simulink model "PID_nn"  (R2018a)
settings: Solver=ode45  StartTime=0.0  StopTime=300  FixedStep=0.001  RelTol=1e-3
undefined symbols (not defined in the file): now
libraries: neural x1, simulink x1
settings Model: Creator=DELL  LastModifiedBy=DELL
settings DataIOCC: ReturnWorkspaceOutputs=on
settings SFSimCC: SimUseLocalCustomCode=on
settings RTWCC: RTWUseLocalCustomCode=on

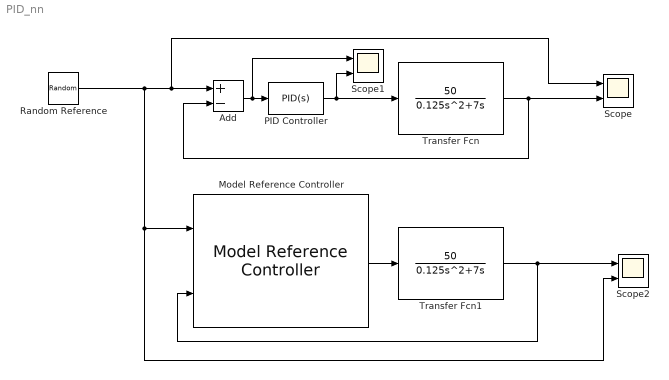
== system PID_nn ==
  Add : Sum  Inputs=+-
  Model Reference Controller : neural/Control Systems/Model Reference Controller  Nrc=2  Nic=1  Njc=2  IW_y=[0.76926837281400406443 1.0491724930046117947;-1.5649571917305367119 -1.6262067418210035541;0.10169527028746853936 -2.2807887773906636575;-0.18348520281428420953 1.7300017256518989139;-1.9381803663322385578 0.68792636179435950883;0.3473292366279158716 -0.31175276926608341821;0.97033314066765130601 -0.86110732257075972562;1.7224524632555133774 0.86294219946467831672;-1.2814965097793364901 -0.73325107298795666466;-1.0971087008827384857 -0.55243059139899131083;0.49228952912381190865 1.9723204963703508952;0.011697439945743900308 0.38975496465121267642;0.83807635467566521381 0.65655305702436839166]  IW_u=[-0.97410868815440343482;-0.78625319749398547842;1.1931167122424097826;2.3091128686597506281;-1.9606186674060903652;1.3783321048282370924;-0.33820842233722908654;0.19846186848270233605;-0.56870285712878521078;-3.408162818861558474;-1.2894532575670551999;-2.4414092268423690513;-1.7602260271262408775]  IW_r=[-0.84197685443253766913 1.7796369390956250367;-0.38707471376110702543 -1.8429755132419081143;-0.16175237051201671323 -0.25342269636000197552;-0.28769428010020853259 0.069271484505792485509;0.70652707134083936324 -0.17276692703880003332;1.0780204878457886331 1.4181813401136305064;-0.051948264329504806325 -1.6445241569225914624;-1.1880960461788905302 1.2154063898199283233;1.1875658765164027741 -0.68921615252562473675;1.5560003500142696176 -0.04350312820646935752;0.44139498586308506534 -1.3033148651935346773;0.18302531326089147012 0.70473704997503994196;1.0523321940101255656 -0.9546522537105888162]  B1_c=[-2.0397585578965609088;-0.89176401210052247404;-0.0029742657793560855518;-0.030720172895946074726;-0.062862692272599107746;0.50457511537373012089;-0.11252509722056680541;-0.17914310024556681644;-1.2510481444352421487;-0.028166471054372609062;-1.7688267194044371422;1.3427849129748476997;2.8761932211087746225]  B2_c=0.37396730159494284695  LW_c=[-0.041043393691476359741 0.019477427718690851904 0.1053907539833678908 -0.73754854177067818988 -1.0246486688178633173 0.22271758836872387888 0.12525474010596918117 0.15647947886094523695 0.014921218230346392983 0.39656411300505045592 -0.015556219376728569817 0.0028930654557257607339 -0.43577395190292017579]  retraining_c=100  max_i_int=2  min_i_int=0.1  max_r_int=2  min_r_int=0.1  Ts=0.05  S1=10  Ni=2  Nj=2  sim_file=PID_  trainfun=trainlm  Use_validation=1  Use_Testing=1  Use_Inc_training=0  Use_previous_weights=1  max_i=0.5  min_i=-0.5  max_r=0.7  min_r=-0.7  sam_training=100  sam_training_c=300  epochs=300  epochs_c=10  minp=-0.35661320607408675265  maxp=0.48591178680951474522  mint=-1.0738732016214509457  maxt=0.48591178680951474522  Normalize=0  IW=[0.67556987563276449382 -0.69678499425169282411;0.00076506828643448034251 -0.0039577200503583681579;0.043175660867651115271 0.011701719069408908491;0.08805266020179439157 -0.061429840952703977652;0.83765129040066044208 -0.26897761024251887196;-0.053575926852162572556 0.054019594938718620836;-0.4029078574550153391 0.41926260157213207647;-0.57774626673100792917 0.57990927253308677258;-0.044816253632694244557 -0.011148646643518222987;-0.058116694762886451919 0.036599082550505646072]  LW1_2=[1.2764114898900797979 -1.3654568303675165275;0.88975936689825596559 1.0016627103752915318;0.2007520367235929859 -0.025320832873496710441;0.69090492155632243776 -0.32818703635270413121;-2.5503569277857729425 -4.1928863881920506174;-0.3911792133524185644 0.21660274613739147198;1.5061446066699322177 -1.7820106033469038653;0.58978056593259375884 -0.13797640336330507793;-0.21389009627626312526 0.03042053703849312285;-0.3846039610556922228 0.1784365941968431013]  LW2_1=[-0.012164931411748257373 -7.1764038912617187055e-05 4.3244167734580489793 0.35404439627012768144 -2.6041631154398130871e-06 2.7716762539423585032 0.0018505676380042724704 -7.333474958736587823e-05 -4.4117740633593669486 -2.9030857530626401619]  B1=[8.3454601252240365739;-1.7535408170190898147;0.70258129456750628705;1.994709437285521636;2.8474709954966814784;0.0049937777892650634867;-3.0112070769960861405;-1.320294485433648024;0.89587938991439508563;0.022105711325819572821]  B2=0.25367965777704626351  S1c=13  Limit_output=1  min_output=-1  max_output=1  Ref_file=robotref
      settings: SourceProductBaseCode=NN
  PID Controller : simulink/Continuous/PID Controller  Controller=PID  Form=Parallel  TimeDomain=Continuous-time  SampleTime=-1  IntegratorMethod=Forward Euler  FilterMethod=Forward Euler  ControllerParametersSource=internal  P=10  I=10  D=0.1  UseFilter=on  N=100  TunerSelectOption=Transfer Function Based (PID Tuner App)  InitialConditionSource=internal  InitialConditionForIntegrator=0  InitialConditionForFilter=0  DifferentiatorICPrevScaledInput=0  ExternalReset=none  TrackingMode=off  Kt=1  LimitOutput=off  UpperSaturationLimit=inf  LowerSaturationLimit=-inf  LinearizeAsGain=on  AntiWindupMode=none  Kb=1  POutMin=[]  POutMax=[]  IOutMin=[]  IOutMax=[]  DOutMin=[]  DOutMax=[]  NOutMin=[]  NOutMax=[]  SumOutMin=[]  SumOutMax=[]  SaturationOutMin=[]  SaturationOutMax=[]  PParamMin=[]  PParamMax=[]  IParamMin=[]  IParamMax=[]  DParamMin=[]  DParamMax=[]  NParamMin=[]  NParamMax=[]  KbParamMin=[]  KbParamMax=[]  KtParamMin=[]  KtParamMax=[]  KbOutMin=[]  KbOutMax=[]  KtOutMin=[]  KtOutMax=[]  IntegratorOutMin=[]  IntegratorOutMax=[]  FilterOutMin=[]  FilterOutMax=[]  SumI1OutMin=[]  SumI1OutMax=[]  SumI2OutMin=[]  SumI2OutMax=[]  SumI3OutMin=[]  SumI3OutMax=[]  SumDOutMin=[]  SumDOutMax=[]  DifferentiatorOutMin=[]  DifferentiatorOutMax=[]  FilterDiffOutCoefMin=[]  FilterDiffOutCoefMax=[]  ReciprocalOutMin=[]  ReciprocalOutMax=[]  SumDenOutMin=[]  SumDenOutMax=[]  SumNumOutMin=[]  SumNumOutMax=[]  DivideOutMin=[]  DivideOutMax=[]  IntegratorContinuousStateAttributes=''  IntegratorStateMustResolveToSignalObject=off  IntegratorRTWStateStorageClass=Auto  FilterContinuousStateAttributes=''  FilterStateMustResolveToSignalObject=off  FilterRTWStateStorageClass=Auto
      settings: AttributesFormatString=|
      | P=%<P>
      | I=%<I>
      | D=%<D>
  Random Reference : UniformRandomNumber  Minimum=-0.5  Maximum=0.5  Seed=round(now)  SampleTime=10
  Scope : Scope  NumInputPorts=2
  Scope1 : Scope  NumInputPorts=2
  Scope2 : Scope  NumInputPorts=2
  Transfer Fcn : TransferFcn  Numerator=[50]  Denominator=[0.125 7 0]
  Transfer Fcn1 : TransferFcn  Numerator=[50]  Denominator=[0.125 7 0]
  wires:
  Random Reference/1 -> Scope2/2, Model Reference Controller/1, Scope/1, Add/1
  Add/1 -> Scope1/1, PID Controller/1
  Transfer Fcn/1 -> Scope/2, Add/2
  PID Controller/1 -> Scope1/2, Transfer Fcn/1
  Model Reference Controller/1 -> Transfer Fcn1/1
  Transfer Fcn1/1 -> Scope2/1, Model Reference Controller/2
